simulink model "rx2"  (R2022b)
settings: Solver=FixedStepDiscrete  StartTime=0.0  StopTime=3.3E6  FixedStep=1  RelTol=1e-3  EnableMultiTasking=on
model workspace (MAT data in the model file):
  mwTaskManagerKernelLatency = 0
undefined symbols (not defined in the file or in its folder): Add, jsin, magnitude, rom_pilot_conj_tt, Shift
libraries: hdlsllib x3231, whdlutilities x525, simulink x260, whdlmod x112, whdledac x26, dsphdlmathfun2 x24, commchan3 x1
(part 4 of 59)

== system rx2/process7/OFDM_DEMOD1 ==
  process : Inport
  process_ctrl : Inport  Port=2  OutDataTypeStr=Bus: BUSOFDM1
  Bus Creator : BusCreator  Inputs=8
  Bus Selector : BusSelector  OutputSignals=signal8 (signal 1).valid,signal8 (signal 2).valid,signal8 (signal 3).valid,signal8 (signal 4).valid,signal8 (signal 5).valid,signal8 (signal 6).valid,signal8 (signal 7).valid,signal8 (signal 8).valid
  Demux : Demux  Outputs=8
  Mux : Mux  Inputs=8
  OFDM_demod1 : Subsystem
  OFDM_demod2 : Subsystem
  OFDM_demod3 : Subsystem
  OFDM_demod4 : Subsystem
  OFDM_demod5 : Subsystem
  OFDM_demod6 : Subsystem
  OFDM_demod7 : Subsystem
  OFDM_demod8 : Subsystem
  rxsig : Outport
  Rcrtl_out : Outport  Port=2  OutDataTypeStr=Bus: BUSOFDM1
  wires:
  process_ctrl/1 -> Bus Selector/1
  process/1 -> Demux/1
  Demux/1 -> OFDM_demod1/1(ofdm_sym)
  Demux/2 -> OFDM_demod2/1(ofdm_sym)
  Bus Selector/2 -> OFDM_demod2/2(valid_in)  "<valid>"
  Demux/3 -> OFDM_demod3/1(ofdm_sym)
  Bus Selector/3 -> OFDM_demod3/2(valid_in)  "<valid>"
  Demux/4 -> OFDM_demod4/1(ofdm_sym)
  Bus Selector/4 -> OFDM_demod4/2(valid_in)  "<valid>"
  Bus Selector/5 -> OFDM_demod5/2(valid_in)  "<valid>"
  Bus Selector/6 -> OFDM_demod6/2(valid_in)  "<valid>"
  Bus Selector/7 -> OFDM_demod8/2(valid_in)  "<valid>"
  Bus Selector/8 -> OFDM_demod7/2(valid_in)  "<valid>"
  Demux/5 -> OFDM_demod5/1(ofdm_sym)
  Demux/6 -> OFDM_demod6/1(ofdm_sym)
  Demux/7 -> OFDM_demod8/1(ofdm_sym)
  Demux/8 -> OFDM_demod7/1(ofdm_sym)
  Bus Selector/1 -> OFDM_demod1/2(valid_in)  "<valid>"
  OFDM_demod5/2(ctrl_out) -> Bus Creator/5  "OFDM_ctrl_bf1_process5"
  OFDM_demod2/1(data_out) -> Mux/2
  OFDM_demod7/2(ctrl_out) -> Bus Creator/8  "OFDM_ctrl_bf1_process8"
  OFDM_demod3/1(data_out) -> Mux/3
  OFDM_demod3/2(ctrl_out) -> Bus Creator/3  "OFDM_ctrl_bf1_process3"
  OFDM_demod8/2(ctrl_out) -> Bus Creator/7  "OFDM_ctrl_bf1_process7"
  OFDM_demod5/1(data_out) -> Mux/5
  OFDM_demod1/1(data_out) -> Mux/1
  OFDM_demod2/2(ctrl_out) -> Bus Creator/2  "OFDM_ctrl_bf1_process2"
  OFDM_demod6/2(ctrl_out) -> Bus Creator/6  "OFDM_ctrl_bf1_process6"
  OFDM_demod8/1(data_out) -> Mux/7
  OFDM_demod6/1(data_out) -> Mux/6
  OFDM_demod4/2(ctrl_out) -> Bus Creator/4  "OFDM_ctrl_bf1_process4"
  OFDM_demod1/2(ctrl_out) -> Bus Creator/1  "OFDM_ctrl_bf1_process1"
  OFDM_demod4/1(data_out) -> Mux/4
  OFDM_demod7/1(data_out) -> Mux/8
  Mux/1 -> rxsig/1
  Bus Creator/1 -> Rcrtl_out/1

== system rx2/process7/decoder ==
  chan_est_tt1 : Inport
  port1_ctrl : Inport  Port=2  OutDataTypeStr=Bus: BUSOFDM1
  rxSig_tt1 : Inport  Port=3
  port2_ctrl : Inport  Port=4  OutDataTypeStr=Bus: BUSOFDM1
  nVar_tt : Inport  Port=5  OutDataTypeStr=fixdt(0,16,12)
  Constant2 : Constant  OutDataTypeStr=boolean
  Constant3 : Constant  Value=72  OutDataTypeStr=uint16
  Delay1 : Delay  InitialCondition=0
  Delay2 : Delay  InitialCondition=0
  Detect Rise Positive : hdlsllib/Logic and Bit Operations/Detect Rise Positive  vinit=0  OutDataTypeStr=boolean
  Detect Rise Positive1 : hdlsllib/Logic and Bit Operations/Detect Rise Positive  vinit=0  OutDataTypeStr=boolean
  MRC : Subsystem
  NR CRC Decoder : whdledac/NR CRC Decoder  CRCType=CRC16  FullCheckSum=on  EnableCRCMaskPort=off  SimulateUsing=Code generation
  NR LDPC Decoder : whdledac/NR LDPC Decoder  Algorithm=Min-sum  ScalingFactor=0.75  Termination=Max  SpecifyInputs=Property  NumIterations=15  MaxNumIterations=30  RateCompatible=off  ParityCheckStatus=off  SimulateUsing=Code generation
  Sample Control Bus Selector1 : whdlutilities/Sample Control Bus Selector  OutputSignals=start,end,valid
  deinterleave : Subsystem  mask{length=1584}
      mask prompts: length "the length of data_in"
      mask DialogControl ParameterGroupVar Prompt: 参数
      mask DialogControl Control2 Prompt: the lantency is (length/2+3)
  p-p : Subsystem
  rate recover : Subsystem
  s-p : Subsystem
  soft demodule : Subsystem  mask{demod_length=1584}
      mask prompts: demod_length "The length of demod"
      mask DialogControl ParameterGroupVar Prompt: 参数
      mask DialogControl Control2 Prompt: Latency=4
  synchronization : Subsystem
  synchronize_valid : Subsystem  mask{valid_length=792}
      mask prompts: valid_length "The length of valid"
      mask DialogControl Control2 Prompt: Latency=2
  data_out : Outport
  valid_out : Outport  Port=2
  wires:
  s-p/2(ctrl_out) -> NR LDPC Decoder/2  "ldpc_in_ctrl"
  p-p/1(data) -> NR CRC Decoder/1  "crc_in"
  p-p/2(ctrl) -> NR CRC Decoder/2  "crc_in_ctrl"
  deinterleave/1(data_out) -> rate recover/1(demod)  "deinterleave_data"
  NR LDPC Decoder/2 -> Sample Control Bus Selector1/1  "ldpc_out_ctrl"
  NR LDPC Decoder/1 -> p-p/1(data_in)  "ldpc_out"
  rate recover/1(rate_recover) -> s-p/1(data_in)  "rm_out"
  Detect Rise Positive/1 -> rate recover/3(start_in)
  s-p/1(data_out) -> NR LDPC Decoder/1  "ldpc_in"
  Sample Control Bus Selector1/1 -> p-p/2(start_in)
  Sample Control Bus Selector1/3 -> p-p/3(valid)
  rate recover/4(valid_out) -> s-p/2(valid_in)  "rm_out_valid"
  Constant3/1 -> NR LDPC Decoder/4
  Constant2/1 -> NR LDPC Decoder/3
  deinterleave/2(valid_out) -> rate recover/2(valid_in), Detect Rise Positive/1  "deinterleave_valid"
  synchronization/1(port1_syn) -> Delay2/1
  synchronization/2(port2_syn) -> Delay1/1
  port2_ctrl/1 -> synchronization/4(port2_ctrl)
  rxSig_tt1/1 -> synchronization/2(rxSig_tt)
  port1_ctrl/1 -> synchronization/3(port1_ctrl)
  chan_est_tt1/1 -> synchronization/1(chan_est_tt)
  synchronization/3(valid_syn) -> Detect Rise Positive1/1
  Detect Rise Positive1/1 -> synchronize_valid/1(start)
  Delay2/1 -> MRC/1(chan_est_tt)  "port1"
  Delay1/1 -> MRC/2(rxSig_tt)  "port2"
  synchronize_valid/1(valid_out) -> MRC/3(valid_tt)  "synchronize_valid"
  nVar_tt/1 -> soft demodule/1(nVar_tt)
  MRC/1(G_k_1) -> soft demodule/2(G_k_1)  "G_k_1"
  MRC/2(r_k) -> soft demodule/3(r_k)  "r_k"
  MRC/4(valid) -> soft demodule/5(valid)
  soft demodule/1(demod) -> deinterleave/1(data_tt)  "demod"
  soft demodule/2(valid_out) -> deinterleave/2(valid_tt)  "valid_in"
  MRC/3(start) -> soft demodule/4(start)
  NR CRC Decoder/1 -> data_out/1  "final_data"
  NR CRC Decoder/2 -> valid_out/1  "final_ctrl"

== system rx2/process8/OFDM_DEMOD1 ==
  process : Inport
  process_ctrl : Inport  Port=2  OutDataTypeStr=Bus: BUSOFDM1
  Bus Creator : BusCreator  Inputs=8
  Bus Selector : BusSelector  OutputSignals=signal9 (signal 1).valid,signal9 (signal 2).valid,signal9 (signal 3).valid,signal9 (signal 4).valid,signal9 (signal 5).valid,signal9 (signal 6).valid,signal9 (signal 7).valid,signal9 (signal 8).valid
  Demux : Demux  Outputs=8
  Mux : Mux  Inputs=8
  OFDM_demod1 : Subsystem
  OFDM_demod2 : Subsystem
  OFDM_demod3 : Subsystem
  OFDM_demod4 : Subsystem
  OFDM_demod5 : Subsystem
  OFDM_demod6 : Subsystem
  OFDM_demod7 : Subsystem
  OFDM_demod8 : Subsystem
  rxsig : Outport
  Rcrtl_out : Outport  Port=2  OutDataTypeStr=Bus: BUSOFDM1
  wires:
  Bus Creator/1 -> Rcrtl_out/1
  Mux/1 -> rxsig/1
  OFDM_demod7/1(data_out) -> Mux/8
  OFDM_demod4/1(data_out) -> Mux/4
  OFDM_demod1/2(ctrl_out) -> Bus Creator/1  "OFDM_ctrl_bf1_process1"
  OFDM_demod4/2(ctrl_out) -> Bus Creator/4  "OFDM_ctrl_bf1_process4"
  OFDM_demod6/1(data_out) -> Mux/6
  OFDM_demod8/1(data_out) -> Mux/7
  OFDM_demod6/2(ctrl_out) -> Bus Creator/6  "OFDM_ctrl_bf1_process6"
  OFDM_demod2/2(ctrl_out) -> Bus Creator/2  "OFDM_ctrl_bf1_process2"
  OFDM_demod1/1(data_out) -> Mux/1
  OFDM_demod5/1(data_out) -> Mux/5
  OFDM_demod8/2(ctrl_out) -> Bus Creator/7  "OFDM_ctrl_bf1_process7"
  OFDM_demod3/2(ctrl_out) -> Bus Creator/3  "OFDM_ctrl_bf1_process3"
  OFDM_demod3/1(data_out) -> Mux/3
  OFDM_demod7/2(ctrl_out) -> Bus Creator/8  "OFDM_ctrl_bf1_process8"
  OFDM_demod2/1(data_out) -> Mux/2
  OFDM_demod5/2(ctrl_out) -> Bus Creator/5  "OFDM_ctrl_bf1_process5"
  Bus Selector/1 -> OFDM_demod1/2(valid_in)  "<valid>"
  Demux/8 -> OFDM_demod7/1(ofdm_sym)
  Demux/7 -> OFDM_demod8/1(ofdm_sym)
  Demux/6 -> OFDM_demod6/1(ofdm_sym)
  Demux/5 -> OFDM_demod5/1(ofdm_sym)
  Bus Selector/8 -> OFDM_demod7/2(valid_in)  "<valid>"
  Bus Selector/7 -> OFDM_demod8/2(valid_in)  "<valid>"
  Bus Selector/6 -> OFDM_demod6/2(valid_in)  "<valid>"
  Bus Selector/5 -> OFDM_demod5/2(valid_in)  "<valid>"
  Bus Selector/4 -> OFDM_demod4/2(valid_in)  "<valid>"
  Demux/4 -> OFDM_demod4/1(ofdm_sym)
  Bus Selector/3 -> OFDM_demod3/2(valid_in)  "<valid>"
  Demux/3 -> OFDM_demod3/1(ofdm_sym)
  Bus Selector/2 -> OFDM_demod2/2(valid_in)  "<valid>"
  Demux/2 -> OFDM_demod2/1(ofdm_sym)
  Demux/1 -> OFDM_demod1/1(ofdm_sym)
  process/1 -> Demux/1
  process_ctrl/1 -> Bus Selector/1

== system rx2/process8/decoder ==
  chan_est_tt1 : Inport
  port1_ctrl : Inport  Port=2  OutDataTypeStr=Bus: BUSOFDM1
  rxSig_tt1 : Inport  Port=3
  port2_ctrl : Inport  Port=4  OutDataTypeStr=Bus: BUSOFDM1
  nVar_tt : Inport  Port=5  OutDataTypeStr=fixdt(0,16,12)
  Constant2 : Constant  OutDataTypeStr=boolean
  Constant3 : Constant  Value=72  OutDataTypeStr=uint16
  Delay1 : Delay  InitialCondition=0
  Delay2 : Delay  InitialCondition=0
  Detect Rise Positive : hdlsllib/Logic and Bit Operations/Detect Rise Positive  vinit=0  OutDataTypeStr=boolean
  Detect Rise Positive1 : hdlsllib/Logic and Bit Operations/Detect Rise Positive  vinit=0  OutDataTypeStr=boolean
  MRC : Subsystem
  NR CRC Decoder : whdledac/NR CRC Decoder  CRCType=CRC16  FullCheckSum=on  EnableCRCMaskPort=off  SimulateUsing=Code generation
  NR LDPC Decoder : whdledac/NR LDPC Decoder  Algorithm=Min-sum  ScalingFactor=0.75  Termination=Max  SpecifyInputs=Property  NumIterations=15  MaxNumIterations=30  RateCompatible=off  ParityCheckStatus=off  SimulateUsing=Code generation
  Sample Control Bus Selector1 : whdlutilities/Sample Control Bus Selector  OutputSignals=start,end,valid
  deinterleave : Subsystem  mask{length=1584}
      mask prompts: length "the length of data_in"
      mask DialogControl ParameterGroupVar Prompt: 参数
      mask DialogControl Control2 Prompt: the lantency is (length/2+3)
  p-p : Subsystem
  rate recover : Subsystem
  s-p : Subsystem
  soft demodule : Subsystem  mask{demod_length=1584}
      mask prompts: demod_length "The length of demod"
      mask DialogControl ParameterGroupVar Prompt: 参数
      mask DialogControl Control2 Prompt: Latency=4
  synchronization : Subsystem
  synchronize_valid : Subsystem  mask{valid_length=792}
      mask prompts: valid_length "The length of valid"
      mask DialogControl Control2 Prompt: Latency=2
  data_out : Outport
  valid_out : Outport  Port=2
  wires:
  NR CRC Decoder/2 -> valid_out/1  "final_ctrl"
  NR CRC Decoder/1 -> data_out/1  "final_data"
  MRC/3(start) -> soft demodule/4(start)
  soft demodule/2(valid_out) -> deinterleave/2(valid_tt)  "valid_in"
  soft demodule/1(demod) -> deinterleave/1(data_tt)  "demod"
  MRC/4(valid) -> soft demodule/5(valid)
  MRC/2(r_k) -> soft demodule/3(r_k)  "r_k"
  MRC/1(G_k_1) -> soft demodule/2(G_k_1)  "G_k_1"
  nVar_tt/1 -> soft demodule/1(nVar_tt)
  synchronize_valid/1(valid_out) -> MRC/3(valid_tt)  "synchronize_valid"
  Delay1/1 -> MRC/2(rxSig_tt)  "port2"
  Delay2/1 -> MRC/1(chan_est_tt)  "port1"
  Detect Rise Positive1/1 -> synchronize_valid/1(start)
  synchronization/3(valid_syn) -> Detect Rise Positive1/1
  chan_est_tt1/1 -> synchronization/1(chan_est_tt)
  port1_ctrl/1 -> synchronization/3(port1_ctrl)
  rxSig_tt1/1 -> synchronization/2(rxSig_tt)
  port2_ctrl/1 -> synchronization/4(port2_ctrl)
  synchronization/2(port2_syn) -> Delay1/1
  synchronization/1(port1_syn) -> Delay2/1
  deinterleave/2(valid_out) -> Detect Rise Positive/1, rate recover/2(valid_in)  "deinterleave_valid"
  Constant2/1 -> NR LDPC Decoder/3
  Constant3/1 -> NR LDPC Decoder/4
  rate recover/4(valid_out) -> s-p/2(valid_in)  "rm_out_valid"
  Sample Control Bus Selector1/3 -> p-p/3(valid)
  Sample Control Bus Selector1/1 -> p-p/2(start_in)
  s-p/1(data_out) -> NR LDPC Decoder/1  "ldpc_in"
  Detect Rise Positive/1 -> rate recover/3(start_in)
  rate recover/1(rate_recover) -> s-p/1(data_in)  "rm_out"
  NR LDPC Decoder/1 -> p-p/1(data_in)  "ldpc_out"
  NR LDPC Decoder/2 -> Sample Control Bus Selector1/1  "ldpc_out_ctrl"
  deinterleave/1(data_out) -> rate recover/1(demod)  "deinterleave_data"
  p-p/2(ctrl) -> NR CRC Decoder/2  "crc_in_ctrl"
  p-p/1(data) -> NR CRC Decoder/1  "crc_in"
  s-p/2(ctrl_out) -> NR LDPC Decoder/2  "ldpc_in_ctrl"

== system rx2/process9/OFDM_DEMOD1 ==
  process : Inport
  process_ctrl : Inport  Port=2  OutDataTypeStr=Bus: BUSOFDM1
  Bus Creator : BusCreator  Inputs=8
  Bus Selector : BusSelector  OutputSignals=signal10 (signal 1).valid,signal10 (signal 2).valid,signal10 (signal 3).valid,signal10 (signal 4).valid,signal10 (signal 5).valid,signal10 (signal 6).valid,signal10 (signal 7).valid,signal10 (signal 8).valid
  Demux : Demux  Outputs=8
  Mux : Mux  Inputs=8
  OFDM_demod1 : Subsystem
  OFDM_demod2 : Subsystem
  OFDM_demod3 : Subsystem
  OFDM_demod4 : Subsystem
  OFDM_demod5 : Subsystem
  OFDM_demod6 : Subsystem
  OFDM_demod7 : Subsystem
  OFDM_demod8 : Subsystem
  rxsig : Outport
  Rcrtl_out : Outport  Port=2  OutDataTypeStr=Bus: BUSOFDM1
  wires:
  process_ctrl/1 -> Bus Selector/1
  process/1 -> Demux/1
  Demux/1 -> OFDM_demod1/1(ofdm_sym)
  Demux/2 -> OFDM_demod2/1(ofdm_sym)
  Bus Selector/2 -> OFDM_demod2/2(valid_in)  "<valid>"
  Demux/3 -> OFDM_demod3/1(ofdm_sym)
  Bus Selector/3 -> OFDM_demod3/2(valid_in)  "<valid>"
  Demux/4 -> OFDM_demod4/1(ofdm_sym)
  Bus Selector/4 -> OFDM_demod4/2(valid_in)  "<valid>"
  Bus Selector/5 -> OFDM_demod5/2(valid_in)  "<valid>"
  Bus Selector/6 -> OFDM_demod6/2(valid_in)  "<valid>"
  Bus Selector/7 -> OFDM_demod8/2(valid_in)  "<valid>"
  Bus Selector/8 -> OFDM_demod7/2(valid_in)  "<valid>"
  Demux/5 -> OFDM_demod5/1(ofdm_sym)
  Demux/6 -> OFDM_demod6/1(ofdm_sym)
  Demux/7 -> OFDM_demod8/1(ofdm_sym)
  Demux/8 -> OFDM_demod7/1(ofdm_sym)
  Bus Selector/1 -> OFDM_demod1/2(valid_in)  "<valid>"
  OFDM_demod5/2(ctrl_out) -> Bus Creator/5  "OFDM_ctrl_bf1_process5"
  OFDM_demod2/1(data_out) -> Mux/2
  OFDM_demod7/2(ctrl_out) -> Bus Creator/8  "OFDM_ctrl_bf1_process8"
  OFDM_demod3/1(data_out) -> Mux/3
  OFDM_demod3/2(ctrl_out) -> Bus Creator/3  "OFDM_ctrl_bf1_process3"
  OFDM_demod8/2(ctrl_out) -> Bus Creator/7  "OFDM_ctrl_bf1_process7"
  OFDM_demod5/1(data_out) -> Mux/5
  OFDM_demod1/1(data_out) -> Mux/1
  OFDM_demod2/2(ctrl_out) -> Bus Creator/2  "OFDM_ctrl_bf1_process2"
  OFDM_demod6/2(ctrl_out) -> Bus Creator/6  "OFDM_ctrl_bf1_process6"
  OFDM_demod8/1(data_out) -> Mux/7
  OFDM_demod6/1(data_out) -> Mux/6
  OFDM_demod4/2(ctrl_out) -> Bus Creator/4  "OFDM_ctrl_bf1_process4"
  OFDM_demod1/2(ctrl_out) -> Bus Creator/1  "OFDM_ctrl_bf1_process1"
  OFDM_demod4/1(data_out) -> Mux/4
  OFDM_demod7/1(data_out) -> Mux/8
  Mux/1 -> rxsig/1
  Bus Creator/1 -> Rcrtl_out/1

== system rx2/process9/decoder ==
  chan_est_tt1 : Inport
  port1_ctrl : Inport  Port=2  OutDataTypeStr=Bus: BUSOFDM1
  rxSig_tt1 : Inport  Port=3
  port2_ctrl : Inport  Port=4  OutDataTypeStr=Bus: BUSOFDM1
  nVar_tt : Inport  Port=5  OutDataTypeStr=fixdt(0,16,12)
  Constant2 : Constant  OutDataTypeStr=boolean
  Constant3 : Constant  Value=72  OutDataTypeStr=uint16
  Delay1 : Delay  InitialCondition=0
  Delay2 : Delay  InitialCondition=0
  Detect Rise Positive : hdlsllib/Logic and Bit Operations/Detect Rise Positive  vinit=0  OutDataTypeStr=boolean
  Detect Rise Positive1 : hdlsllib/Logic and Bit Operations/Detect Rise Positive  vinit=0  OutDataTypeStr=boolean
  MRC : Subsystem
  NR CRC Decoder : whdledac/NR CRC Decoder  CRCType=CRC16  FullCheckSum=on  EnableCRCMaskPort=off  SimulateUsing=Code generation
  NR LDPC Decoder : whdledac/NR LDPC Decoder  Algorithm=Min-sum  ScalingFactor=0.75  Termination=Max  SpecifyInputs=Property  NumIterations=15  MaxNumIterations=30  RateCompatible=off  ParityCheckStatus=off  SimulateUsing=Code generation
  Sample Control Bus Selector1 : whdlutilities/Sample Control Bus Selector  OutputSignals=start,end,valid
  deinterleave : Subsystem  mask{length=1584}
      mask prompts: length "the length of data_in"
      mask DialogControl ParameterGroupVar Prompt: 参数
      mask DialogControl Control2 Prompt: the lantency is (length/2+3)
  p-p : Subsystem
  rate recover : Subsystem
  s-p : Subsystem
  soft demodule : Subsystem  mask{demod_length=1584}
      mask prompts: demod_length "The length of demod"
      mask DialogControl ParameterGroupVar Prompt: 参数
      mask DialogControl Control2 Prompt: Latency=4
  synchronization : Subsystem
  synchronize_valid : Subsystem  mask{valid_length=792}
      mask prompts: valid_length "The length of valid"
      mask DialogControl Control2 Prompt: Latency=2
  data_out : Outport
  valid_out : Outport  Port=2
  wires:
  s-p/2(ctrl_out) -> NR LDPC Decoder/2  "ldpc_in_ctrl"
  p-p/1(data) -> NR CRC Decoder/1  "crc_in"
  p-p/2(ctrl) -> NR CRC Decoder/2  "crc_in_ctrl"
  deinterleave/1(data_out) -> rate recover/1(demod)  "deinterleave_data"
  NR LDPC Decoder/2 -> Sample Control Bus Selector1/1  "ldpc_out_ctrl"
  NR LDPC Decoder/1 -> p-p/1(data_in)  "ldpc_out"
  rate recover/1(rate_recover) -> s-p/1(data_in)  "rm_out"
  Detect Rise Positive/1 -> rate recover/3(start_in)
  s-p/1(data_out) -> NR LDPC Decoder/1  "ldpc_in"
  Sample Control Bus Selector1/1 -> p-p/2(start_in)
  Sample Control Bus Selector1/3 -> p-p/3(valid)
  rate recover/4(valid_out) -> s-p/2(valid_in)  "rm_out_valid"
  Constant3/1 -> NR LDPC Decoder/4
  Constant2/1 -> NR LDPC Decoder/3
  deinterleave/2(valid_out) -> rate recover/2(valid_in), Detect Rise Positive/1  "deinterleave_valid"
  synchronization/1(port1_syn) -> Delay2/1
  synchronization/2(port2_syn) -> Delay1/1
  port2_ctrl/1 -> synchronization/4(port2_ctrl)
  rxSig_tt1/1 -> synchronization/2(rxSig_tt)
  port1_ctrl/1 -> synchronization/3(port1_ctrl)
  chan_est_tt1/1 -> synchronization/1(chan_est_tt)
  synchronization/3(valid_syn) -> Detect Rise Positive1/1
  Detect Rise Positive1/1 -> synchronize_valid/1(start)
  Delay2/1 -> MRC/1(chan_est_tt)  "port1"
  Delay1/1 -> MRC/2(rxSig_tt)  "port2"
  synchronize_valid/1(valid_out) -> MRC/3(valid_tt)  "synchronize_valid"
  nVar_tt/1 -> soft demodule/1(nVar_tt)
  MRC/1(G_k_1) -> soft demodule/2(G_k_1)  "G_k_1"
  MRC/2(r_k) -> soft demodule/3(r_k)  "r_k"
  MRC/4(valid) -> soft demodule/5(valid)
  soft demodule/1(demod) -> deinterleave/1(data_tt)  "demod"
  soft demodule/2(valid_out) -> deinterleave/2(valid_tt)  "valid_in"
  MRC/3(start) -> soft demodule/4(start)
  NR CRC Decoder/1 -> data_out/1  "final_data"
  NR CRC Decoder/2 -> valid_out/1  "final_ctrl"

== system rx2/demode1/chan_est1/Subsystem ==
  data_in : Inport
  ctrl_in : Inport  Port=2  OutDataTypeStr=Bus: BUSOFDM1
  HDL_DUT : Subsystem
  HDL_DUT1 : Subsystem
  HDL_DUT2 : Subsystem
  HDL_DUT3 : Subsystem
  HDL_DUT4 : Subsystem
  HDL_DUT5 : Subsystem
  HDL_DUT6 : Subsystem
  HDL_DUT7 : Subsystem
  OFDM_DEMOD1 : Subsystem
  Subsystem1 : Subsystem
  H_out : Outport
  crtl_out : Outport  Port=2  OutDataTypeStr=Bus: BUSOFDM1
  σ²_out : Outport  Port=3
  wires:
  Subsystem1/1(Out1) -> H_out/1
  Subsystem1/3(σ²) -> σ²_out/1
  Subsystem1/2(Out3) -> crtl_out/1
  HDL_DUT/2(w_out) -> Subsystem1/2(w_out)  "w_out"
  HDL_DUT/3(ctrl_out) -> Subsystem1/3(In3)
  HDL_DUT/1(H_out) -> Subsystem1/1(H_out)  "H_out"
  data_in/1 -> OFDM_DEMOD1/1(process)
  OFDM_DEMOD1/1(data_in) -> HDL_DUT/1(data_in)
  ctrl_in/1 -> OFDM_DEMOD1/2(process_ctrl)
  OFDM_DEMOD1/2(OFDM_ctrl_bf1_process1) -> HDL_DUT/2(ctrl_in)
  OFDM_DEMOD1/3(Out3) -> HDL_DUT1/1(data_in)
  OFDM_DEMOD1/4(OFDM_ctrl_bf1_process2) -> HDL_DUT1/2(ctrl_in)
  OFDM_DEMOD1/5(Out5) -> HDL_DUT2/1(data_in)
  OFDM_DEMOD1/6(OFDM_ctrl_bf1_process3) -> HDL_DUT2/2(ctrl_in)
  OFDM_DEMOD1/7(Out7) -> HDL_DUT3/1(data_in)
  OFDM_DEMOD1/8(OFDM_ctrl_bf1_process4) -> HDL_DUT3/2(ctrl_in)
  OFDM_DEMOD1/9(Out9) -> HDL_DUT4/1(data_in)
  OFDM_DEMOD1/10(OFDM_ctrl_bf1_process5) -> HDL_DUT4/2(ctrl_in)
  OFDM_DEMOD1/11(Out11) -> HDL_DUT5/1(data_in)
  OFDM_DEMOD1/12(OFDM_ctrl_bf1_process6) -> HDL_DUT5/2(ctrl_in)
  OFDM_DEMOD1/13(Out13) -> HDL_DUT6/1(data_in)
  OFDM_DEMOD1/14(OFDM_ctrl_bf1_process7) -> HDL_DUT6/2(ctrl_in)
  OFDM_DEMOD1/15(Out15) -> HDL_DUT7/1(data_in)
  OFDM_DEMOD1/16(OFDM_ctrl_bf1_process8) -> HDL_DUT7/2(ctrl_in)
  HDL_DUT1/1(H_out) -> Subsystem1/4(H_out1)  "H_out"
  HDL_DUT1/2(w_out) -> Subsystem1/5(w_out1)  "w_out"
  HDL_DUT1/3(ctrl_out) -> Subsystem1/6(ctrl_out)
  HDL_DUT2/1(H_out) -> Subsystem1/7(H_out2)  "H_out"
  HDL_DUT2/2(w_out) -> Subsystem1/8(w_out2)  "w_out"
  HDL_DUT2/3(ctrl_out) -> Subsystem1/9(In9)
  HDL_DUT3/1(H_out) -> Subsystem1/10(H_out3)  "H_out"
  HDL_DUT3/2(w_out) -> Subsystem1/11(w_out3)  "w_out"
  HDL_DUT3/3(ctrl_out) -> Subsystem1/12(In12)
  HDL_DUT4/1(H_out) -> Subsystem1/13(H_out4)  "H_out"
  HDL_DUT4/2(w_out) -> Subsystem1/14(w_out4)  "w_out"
  HDL_DUT4/3(ctrl_out) -> Subsystem1/15(In15)
  HDL_DUT5/1(H_out) -> Subsystem1/16(H_out5)  "H_out"
  HDL_DUT5/2(w_out) -> Subsystem1/17(w_out5)  "w_out"
  HDL_DUT5/3(ctrl_out) -> Subsystem1/18(In18)
  HDL_DUT6/1(H_out) -> Subsystem1/19(H_out6)  "H_out"
  HDL_DUT6/2(w_out) -> Subsystem1/20(w_out6)  "w_out"
  HDL_DUT6/3(ctrl_out) -> Subsystem1/21(In21)
  HDL_DUT7/1(H_out) -> Subsystem1/22(H_out7)  "H_out"
  HDL_DUT7/2(w_out) -> Subsystem1/23(w_out7)  "w_out"
  HDL_DUT7/3(ctrl_out) -> Subsystem1/24(In24)

== system rx2/process divide/transport_block1/Subsystem1 ==
  data_in : Inport
  select_valid : Inport  Port=2  OutDataTypeStr=boolean
  Constant : Constant  Value=0  OutDataTypeStr=fixdt(1,16,14)
  Real-Imag to Complex : RealImagToComplex
  Switch : Switch  Criteria=u2 ~= 0  SaturateOnIntegerOverflow=off  InputSameDT=off
  ctrl_gen : Subsystem
  data_out : Outport
  ctrl_out : Outport  Port=2
  wires:
  Switch/1 -> ctrl_gen/1(data_in)
  Constant/1 -> Real-Imag to Complex/2, Real-Imag to Complex/1
  select_valid/1 -> ctrl_gen/2(valid_in), Switch/2
  ctrl_gen/1(data_out) -> data_out/1
  ctrl_gen/2(ctrl_out) -> ctrl_out/1
  data_in/1 -> Switch/1
  Real-Imag to Complex/1 -> Switch/3

== system rx2/process divide/transport_block1/Subsystem10 ==
  data_in : Inport
  select_valid : Inport  Port=2  OutDataTypeStr=boolean
  Constant : Constant  Value=0  OutDataTypeStr=fixdt(1,16,14)
  Real-Imag to Complex : RealImagToComplex
  Switch : Switch  Criteria=u2 ~= 0  SaturateOnIntegerOverflow=off  InputSameDT=off
  ctrl_gen : Subsystem
  data_out : Outport
  ctrl_out : Outport  Port=2
  wires:
  Real-Imag to Complex/1 -> Switch/3
  data_in/1 -> Switch/1
  ctrl_gen/2(ctrl_out) -> ctrl_out/1
  ctrl_gen/1(data_out) -> data_out/1
  select_valid/1 -> Switch/2, ctrl_gen/2(valid_in)
  Constant/1 -> Real-Imag to Complex/1, Real-Imag to Complex/2
  Switch/1 -> ctrl_gen/1(data_in)

== system rx2/process divide/transport_block1/Subsystem11 ==
  data_in : Inport
  select_valid : Inport  Port=2  OutDataTypeStr=boolean
  Constant : Constant  Value=0  OutDataTypeStr=fixdt(1,16,14)
  Real-Imag to Complex : RealImagToComplex
  Switch : Switch  Criteria=u2 ~= 0  SaturateOnIntegerOverflow=off  InputSameDT=off
  ctrl_gen : Subsystem
  data_out : Outport
  ctrl_out : Outport  Port=2
  wires:
  Real-Imag to Complex/1 -> Switch/3
  data_in/1 -> Switch/1
  ctrl_gen/2(ctrl_out) -> ctrl_out/1
  ctrl_gen/1(data_out) -> data_out/1
  select_valid/1 -> Switch/2, ctrl_gen/2(valid_in)
  Constant/1 -> Real-Imag to Complex/1, Real-Imag to Complex/2
  Switch/1 -> ctrl_gen/1(data_in)

== system rx2/process divide/transport_block1/Subsystem12 ==
  data_in : Inport
  select_valid : Inport  Port=2  OutDataTypeStr=boolean
  Constant : Constant  Value=0  OutDataTypeStr=fixdt(1,16,14)
  Real-Imag to Complex : RealImagToComplex
  Switch : Switch  Criteria=u2 ~= 0  SaturateOnIntegerOverflow=off  InputSameDT=off
  ctrl_gen : Subsystem
  data_out : Outport
  ctrl_out : Outport  Port=2
  wires:
  Real-Imag to Complex/1 -> Switch/3
  data_in/1 -> Switch/1
  ctrl_gen/2(ctrl_out) -> ctrl_out/1
  ctrl_gen/1(data_out) -> data_out/1
  select_valid/1 -> Switch/2, ctrl_gen/2(valid_in)
  Constant/1 -> Real-Imag to Complex/1, Real-Imag to Complex/2
  Switch/1 -> ctrl_gen/1(data_in)

== system rx2/process divide/transport_block1/Subsystem13 ==
  data_in : Inport
  select_valid : Inport  Port=2  OutDataTypeStr=boolean
  Constant : Constant  Value=0  OutDataTypeStr=fixdt(1,16,14)
  Real-Imag to Complex : RealImagToComplex
  Switch : Switch  Criteria=u2 ~= 0  SaturateOnIntegerOverflow=off  InputSameDT=off
  ctrl_gen : Subsystem
  data_out : Outport
  ctrl_out : Outport  Port=2
  wires:
  Real-Imag to Complex/1 -> Switch/3
  data_in/1 -> Switch/1
  ctrl_gen/2(ctrl_out) -> ctrl_out/1
  ctrl_gen/1(data_out) -> data_out/1
  select_valid/1 -> Switch/2, ctrl_gen/2(valid_in)
  Constant/1 -> Real-Imag to Complex/1, Real-Imag to Complex/2
  Switch/1 -> ctrl_gen/1(data_in)

== system rx2/process divide/transport_block1/Subsystem14 ==
  data_in : Inport
  select_valid : Inport  Port=2  OutDataTypeStr=boolean
  Constant : Constant  Value=0  OutDataTypeStr=fixdt(1,16,14)
  Real-Imag to Complex : RealImagToComplex
  Switch : Switch  Criteria=u2 ~= 0  SaturateOnIntegerOverflow=off  InputSameDT=off
  ctrl_gen : Subsystem
  data_out : Outport
  ctrl_out : Outport  Port=2
  wires:
  Real-Imag to Complex/1 -> Switch/3
  data_in/1 -> Switch/1
  ctrl_gen/2(ctrl_out) -> ctrl_out/1
  ctrl_gen/1(data_out) -> data_out/1
  select_valid/1 -> Switch/2, ctrl_gen/2(valid_in)
  Constant/1 -> Real-Imag to Complex/1, Real-Imag to Complex/2
  Switch/1 -> ctrl_gen/1(data_in)

== system rx2/process divide/transport_block1/Subsystem2 ==
  data_in : Inport
  select_valid : Inport  Port=2  OutDataTypeStr=boolean
  Constant : Constant  Value=0  OutDataTypeStr=fixdt(1,16,14)
  Real-Imag to Complex : RealImagToComplex
  Switch : Switch  Criteria=u2 ~= 0  SaturateOnIntegerOverflow=off  InputSameDT=off
  ctrl_gen : Subsystem
  data_out : Outport
  ctrl_out : Outport  Port=2
  wires:
  Real-Imag to Complex/1 -> Switch/3
  data_in/1 -> Switch/1
  ctrl_gen/2(ctrl_out) -> ctrl_out/1
  ctrl_gen/1(data_out) -> data_out/1
  select_valid/1 -> Switch/2, ctrl_gen/2(valid_in)
  Constant/1 -> Real-Imag to Complex/1, Real-Imag to Complex/2
  Switch/1 -> ctrl_gen/1(data_in)

== system rx2/process divide/transport_block1/Subsystem3 ==
  data_in : Inport
  select_valid : Inport  Port=2  OutDataTypeStr=boolean
  Constant : Constant  Value=0  OutDataTypeStr=fixdt(1,16,14)
  Real-Imag to Complex : RealImagToComplex
  Switch : Switch  Criteria=u2 ~= 0  SaturateOnIntegerOverflow=off  InputSameDT=off
  ctrl_gen : Subsystem
  data_out : Outport
  ctrl_out : Outport  Port=2
  wires:
  Switch/1 -> ctrl_gen/1(data_in)
  Constant/1 -> Real-Imag to Complex/2, Real-Imag to Complex/1
  select_valid/1 -> ctrl_gen/2(valid_in), Switch/2
  ctrl_gen/1(data_out) -> data_out/1
  ctrl_gen/2(ctrl_out) -> ctrl_out/1
  data_in/1 -> Switch/1
  Real-Imag to Complex/1 -> Switch/3

== system rx2/process divide/transport_block1/Subsystem4 ==
  data_in : Inport
  select_valid : Inport  Port=2  OutDataTypeStr=boolean
  Constant : Constant  Value=0  OutDataTypeStr=fixdt(1,16,14)
  Real-Imag to Complex : RealImagToComplex
  Switch : Switch  Criteria=u2 ~= 0  SaturateOnIntegerOverflow=off  InputSameDT=off
  ctrl_gen : Subsystem
  data_out : Outport
  ctrl_out : Outport  Port=2
  wires:
  Real-Imag to Complex/1 -> Switch/3
  data_in/1 -> Switch/1
  ctrl_gen/2(ctrl_out) -> ctrl_out/1
  ctrl_gen/1(data_out) -> data_out/1
  select_valid/1 -> Switch/2, ctrl_gen/2(valid_in)
  Constant/1 -> Real-Imag to Complex/1, Real-Imag to Complex/2
  Switch/1 -> ctrl_gen/1(data_in)

== system rx2/process divide/transport_block1/Subsystem5 ==
  data_in : Inport
  select_valid : Inport  Port=2  OutDataTypeStr=boolean
  Constant : Constant  Value=0  OutDataTypeStr=fixdt(1,16,14)
  Real-Imag to Complex : RealImagToComplex
  Switch : Switch  Criteria=u2 ~= 0  SaturateOnIntegerOverflow=off  InputSameDT=off
  ctrl_gen : Subsystem
  data_out : Outport
  ctrl_out : Outport  Port=2
  wires:
  Real-Imag to Complex/1 -> Switch/3
  data_in/1 -> Switch/1
  ctrl_gen/2(ctrl_out) -> ctrl_out/1
  ctrl_gen/1(data_out) -> data_out/1
  select_valid/1 -> Switch/2, ctrl_gen/2(valid_in)
  Constant/1 -> Real-Imag to Complex/1, Real-Imag to Complex/2
  Switch/1 -> ctrl_gen/1(data_in)

== system rx2/process divide/transport_block1/Subsystem6 ==
  data_in : Inport
  select_valid : Inport  Port=2  OutDataTypeStr=boolean
  Constant : Constant  Value=0  OutDataTypeStr=fixdt(1,16,14)
  Real-Imag to Complex : RealImagToComplex
  Switch : Switch  Criteria=u2 ~= 0  SaturateOnIntegerOverflow=off  InputSameDT=off
  ctrl_gen : Subsystem
  data_out : Outport
  ctrl_out : Outport  Port=2
  wires:
  Real-Imag to Complex/1 -> Switch/3
  data_in/1 -> Switch/1
  ctrl_gen/2(ctrl_out) -> ctrl_out/1
  ctrl_gen/1(data_out) -> data_out/1
  select_valid/1 -> Switch/2, ctrl_gen/2(valid_in)
  Constant/1 -> Real-Imag to Complex/1, Real-Imag to Complex/2
  Switch/1 -> ctrl_gen/1(data_in)

== system rx2/process divide/transport_block1/Subsystem7 ==
  data_in : Inport
  select_valid : Inport  Port=2  OutDataTypeStr=boolean
  Constant : Constant  Value=0  OutDataTypeStr=fixdt(1,16,14)
  Real-Imag to Complex : RealImagToComplex
  Switch : Switch  Criteria=u2 ~= 0  SaturateOnIntegerOverflow=off  InputSameDT=off
  ctrl_gen : Subsystem
  data_out : Outport
  ctrl_out : Outport  Port=2
  wires:
  Real-Imag to Complex/1 -> Switch/3
  data_in/1 -> Switch/1
  ctrl_gen/2(ctrl_out) -> ctrl_out/1
  ctrl_gen/1(data_out) -> data_out/1
  select_valid/1 -> Switch/2, ctrl_gen/2(valid_in)
  Constant/1 -> Real-Imag to Complex/1, Real-Imag to Complex/2
  Switch/1 -> ctrl_gen/1(data_in)

== system rx2/process divide/transport_block1/Subsystem8 ==
  data_in : Inport
  select_valid : Inport  Port=2  OutDataTypeStr=boolean
  Constant : Constant  Value=0  OutDataTypeStr=fixdt(1,16,14)
  Real-Imag to Complex : RealImagToComplex
  Switch : Switch  Criteria=u2 ~= 0  SaturateOnIntegerOverflow=off  InputSameDT=off
  ctrl_gen : Subsystem
  data_out : Outport
  ctrl_out : Outport  Port=2
  wires:
  Real-Imag to Complex/1 -> Switch/3
  data_in/1 -> Switch/1
  ctrl_gen/2(ctrl_out) -> ctrl_out/1
  ctrl_gen/1(data_out) -> data_out/1
  select_valid/1 -> Switch/2, ctrl_gen/2(valid_in)
  Constant/1 -> Real-Imag to Complex/1, Real-Imag to Complex/2
  Switch/1 -> ctrl_gen/1(data_in)

== system rx2/process divide/transport_block1/Subsystem9 ==
  data_in : Inport
  select_valid : Inport  Port=2  OutDataTypeStr=boolean
  Constant : Constant  Value=0  OutDataTypeStr=fixdt(1,16,14)
  Real-Imag to Complex : RealImagToComplex
  Switch : Switch  Criteria=u2 ~= 0  SaturateOnIntegerOverflow=off  InputSameDT=off
  ctrl_gen : Subsystem
  data_out : Outport
  ctrl_out : Outport  Port=2
  wires:
  Real-Imag to Complex/1 -> Switch/3
  data_in/1 -> Switch/1
  ctrl_gen/2(ctrl_out) -> ctrl_out/1
  ctrl_gen/1(data_out) -> data_out/1
  select_valid/1 -> Switch/2, ctrl_gen/2(valid_in)
  Constant/1 -> Real-Imag to Complex/1, Real-Imag to Complex/2
  Switch/1 -> ctrl_gen/1(data_in)

== system rx2/process divide/transport_block2/Subsystem1 ==
  data_in : Inport
  select_valid : Inport  Port=2  OutDataTypeStr=boolean
  Constant : Constant  Value=0  OutDataTypeStr=fixdt(1,16,14)
  Real-Imag to Complex : RealImagToComplex
  Switch : Switch  Criteria=u2 ~= 0  SaturateOnIntegerOverflow=off  InputSameDT=off
  ctrl_gen : Subsystem
  data_out : Outport
  ctrl_out : Outport  Port=2
  wires:
  Real-Imag to Complex/1 -> Switch/3
  data_in/1 -> Switch/1
  ctrl_gen/2(ctrl_out) -> ctrl_out/1
  ctrl_gen/1(data_out) -> data_out/1
  select_valid/1 -> Switch/2, ctrl_gen/2(valid_in)
  Constant/1 -> Real-Imag to Complex/1, Real-Imag to Complex/2
  Switch/1 -> ctrl_gen/1(data_in)

== system rx2/process divide/transport_block2/Subsystem10 ==
  data_in : Inport
  select_valid : Inport  Port=2  OutDataTypeStr=boolean
  Constant : Constant  Value=0  OutDataTypeStr=fixdt(1,16,14)
  Real-Imag to Complex : RealImagToComplex
  Switch : Switch  Criteria=u2 ~= 0  SaturateOnIntegerOverflow=off  InputSameDT=off
  ctrl_gen : Subsystem
  data_out : Outport
  ctrl_out : Outport  Port=2
  wires:
  Switch/1 -> ctrl_gen/1(data_in)
  Constant/1 -> Real-Imag to Complex/2, Real-Imag to Complex/1
  select_valid/1 -> ctrl_gen/2(valid_in), Switch/2
  ctrl_gen/1(data_out) -> data_out/1
  ctrl_gen/2(ctrl_out) -> ctrl_out/1
  data_in/1 -> Switch/1
  Real-Imag to Complex/1 -> Switch/3

== system rx2/process divide/transport_block2/Subsystem11 ==
  data_in : Inport
  select_valid : Inport  Port=2  OutDataTypeStr=boolean
  Constant : Constant  Value=0  OutDataTypeStr=fixdt(1,16,14)
  Real-Imag to Complex : RealImagToComplex
  Switch : Switch  Criteria=u2 ~= 0  SaturateOnIntegerOverflow=off  InputSameDT=off
  ctrl_gen : Subsystem
  data_out : Outport
  ctrl_out : Outport  Port=2
  wires:
  Switch/1 -> ctrl_gen/1(data_in)
  Constant/1 -> Real-Imag to Complex/2, Real-Imag to Complex/1
  select_valid/1 -> ctrl_gen/2(valid_in), Switch/2
  ctrl_gen/1(data_out) -> data_out/1
  ctrl_gen/2(ctrl_out) -> ctrl_out/1
  data_in/1 -> Switch/1
  Real-Imag to Complex/1 -> Switch/3

== system rx2/process divide/transport_block2/Subsystem12 ==
  data_in : Inport
  select_valid : Inport  Port=2  OutDataTypeStr=boolean
  Constant : Constant  Value=0  OutDataTypeStr=fixdt(1,16,14)
  Real-Imag to Complex : RealImagToComplex
  Switch : Switch  Criteria=u2 ~= 0  SaturateOnIntegerOverflow=off  InputSameDT=off
  ctrl_gen : Subsystem
  data_out : Outport
  ctrl_out : Outport  Port=2
  wires:
  Switch/1 -> ctrl_gen/1(data_in)
  Constant/1 -> Real-Imag to Complex/2, Real-Imag to Complex/1
  select_valid/1 -> ctrl_gen/2(valid_in), Switch/2
  ctrl_gen/1(data_out) -> data_out/1
  ctrl_gen/2(ctrl_out) -> ctrl_out/1
  data_in/1 -> Switch/1
  Real-Imag to Complex/1 -> Switch/3

== system rx2/process divide/transport_block2/Subsystem13 ==
  data_in : Inport
  select_valid : Inport  Port=2  OutDataTypeStr=boolean
  Constant : Constant  Value=0  OutDataTypeStr=fixdt(1,16,14)
  Real-Imag to Complex : RealImagToComplex
  Switch : Switch  Criteria=u2 ~= 0  SaturateOnIntegerOverflow=off  InputSameDT=off
  ctrl_gen : Subsystem
  data_out : Outport
  ctrl_out : Outport  Port=2
  wires:
  Switch/1 -> ctrl_gen/1(data_in)
  Constant/1 -> Real-Imag to Complex/2, Real-Imag to Complex/1
  select_valid/1 -> ctrl_gen/2(valid_in), Switch/2
  ctrl_gen/1(data_out) -> data_out/1
  ctrl_gen/2(ctrl_out) -> ctrl_out/1
  data_in/1 -> Switch/1
  Real-Imag to Complex/1 -> Switch/3

== system rx2/process divide/transport_block2/Subsystem14 ==
  data_in : Inport
  select_valid : Inport  Port=2  OutDataTypeStr=boolean
  Constant : Constant  Value=0  OutDataTypeStr=fixdt(1,16,14)
  Real-Imag to Complex : RealImagToComplex
  Switch : Switch  Criteria=u2 ~= 0  SaturateOnIntegerOverflow=off  InputSameDT=off
  ctrl_gen : Subsystem
  data_out : Outport
  ctrl_out : Outport  Port=2
  wires:
  Switch/1 -> ctrl_gen/1(data_in)
  Constant/1 -> Real-Imag to Complex/2, Real-Imag to Complex/1
  select_valid/1 -> ctrl_gen/2(valid_in), Switch/2
  ctrl_gen/1(data_out) -> data_out/1
  ctrl_gen/2(ctrl_out) -> ctrl_out/1
  data_in/1 -> Switch/1
  Real-Imag to Complex/1 -> Switch/3

== system rx2/process divide/transport_block2/Subsystem2 ==
  data_in : Inport
  select_valid : Inport  Port=2  OutDataTypeStr=boolean
  Constant : Constant  Value=0  OutDataTypeStr=fixdt(1,16,14)
  Real-Imag to Complex : RealImagToComplex
  Switch : Switch  Criteria=u2 ~= 0  SaturateOnIntegerOverflow=off  InputSameDT=off
  ctrl_gen : Subsystem
  data_out : Outport
  ctrl_out : Outport  Port=2
  wires:
  Switch/1 -> ctrl_gen/1(data_in)
  Constant/1 -> Real-Imag to Complex/2, Real-Imag to Complex/1
  select_valid/1 -> ctrl_gen/2(valid_in), Switch/2
  ctrl_gen/1(data_out) -> data_out/1
  ctrl_gen/2(ctrl_out) -> ctrl_out/1
  data_in/1 -> Switch/1
  Real-Imag to Complex/1 -> Switch/3

== system rx2/process divide/transport_block2/Subsystem3 ==
  data_in : Inport
  select_valid : Inport  Port=2  OutDataTypeStr=boolean
  Constant : Constant  Value=0  OutDataTypeStr=fixdt(1,16,14)
  Real-Imag to Complex : RealImagToComplex
  Switch : Switch  Criteria=u2 ~= 0  SaturateOnIntegerOverflow=off  InputSameDT=off
  ctrl_gen : Subsystem
  data_out : Outport
  ctrl_out : Outport  Port=2
  wires:
  Real-Imag to Complex/1 -> Switch/3
  data_in/1 -> Switch/1
  ctrl_gen/2(ctrl_out) -> ctrl_out/1
  ctrl_gen/1(data_out) -> data_out/1
  select_valid/1 -> Switch/2, ctrl_gen/2(valid_in)
  Constant/1 -> Real-Imag to Complex/1, Real-Imag to Complex/2
  Switch/1 -> ctrl_gen/1(data_in)

== system rx2/process divide/transport_block2/Subsystem4 ==
  data_in : Inport
  select_valid : Inport  Port=2  OutDataTypeStr=boolean
  Constant : Constant  Value=0  OutDataTypeStr=fixdt(1,16,14)
  Real-Imag to Complex : RealImagToComplex
  Switch : Switch  Criteria=u2 ~= 0  SaturateOnIntegerOverflow=off  InputSameDT=off
  ctrl_gen : Subsystem
  data_out : Outport
  ctrl_out : Outport  Port=2
  wires:
  Switch/1 -> ctrl_gen/1(data_in)
  Constant/1 -> Real-Imag to Complex/2, Real-Imag to Complex/1
  select_valid/1 -> ctrl_gen/2(valid_in), Switch/2
  ctrl_gen/1(data_out) -> data_out/1
  ctrl_gen/2(ctrl_out) -> ctrl_out/1
  data_in/1 -> Switch/1
  Real-Imag to Complex/1 -> Switch/3

== system rx2/process divide/transport_block2/Subsystem5 ==
  data_in : Inport
  select_valid : Inport  Port=2  OutDataTypeStr=boolean
  Constant : Constant  Value=0  OutDataTypeStr=fixdt(1,16,14)
  Real-Imag to Complex : RealImagToComplex
  Switch : Switch  Criteria=u2 ~= 0  SaturateOnIntegerOverflow=off  InputSameDT=off
  ctrl_gen : Subsystem
  data_out : Outport
  ctrl_out : Outport  Port=2
  wires:
  Switch/1 -> ctrl_gen/1(data_in)
  Constant/1 -> Real-Imag to Complex/2, Real-Imag to Complex/1
  select_valid/1 -> ctrl_gen/2(valid_in), Switch/2
  ctrl_gen/1(data_out) -> data_out/1
  ctrl_gen/2(ctrl_out) -> ctrl_out/1
  data_in/1 -> Switch/1
  Real-Imag to Complex/1 -> Switch/3

== system rx2/process divide/transport_block2/Subsystem6 ==
  data_in : Inport
  select_valid : Inport  Port=2  OutDataTypeStr=boolean
  Constant : Constant  Value=0  OutDataTypeStr=fixdt(1,16,14)
  Real-Imag to Complex : RealImagToComplex
  Switch : Switch  Criteria=u2 ~= 0  SaturateOnIntegerOverflow=off  InputSameDT=off
  ctrl_gen : Subsystem
  data_out : Outport
  ctrl_out : Outport  Port=2
  wires:
  Switch/1 -> ctrl_gen/1(data_in)
  Constant/1 -> Real-Imag to Complex/2, Real-Imag to Complex/1
  select_valid/1 -> ctrl_gen/2(valid_in), Switch/2
  ctrl_gen/1(data_out) -> data_out/1
  ctrl_gen/2(ctrl_out) -> ctrl_out/1
  data_in/1 -> Switch/1
  Real-Imag to Complex/1 -> Switch/3

== system rx2/process divide/transport_block2/Subsystem7 ==
  data_in : Inport
  select_valid : Inport  Port=2  OutDataTypeStr=boolean
  Constant : Constant  Value=0  OutDataTypeStr=fixdt(1,16,14)
  Real-Imag to Complex : RealImagToComplex
  Switch : Switch  Criteria=u2 ~= 0  SaturateOnIntegerOverflow=off  InputSameDT=off
  ctrl_gen : Subsystem
  data_out : Outport
  ctrl_out : Outport  Port=2
  wires:
  Switch/1 -> ctrl_gen/1(data_in)
  Constant/1 -> Real-Imag to Complex/2, Real-Imag to Complex/1
  select_valid/1 -> ctrl_gen/2(valid_in), Switch/2
  ctrl_gen/1(data_out) -> data_out/1
  ctrl_gen/2(ctrl_out) -> ctrl_out/1
  data_in/1 -> Switch/1
  Real-Imag to Complex/1 -> Switch/3

== system rx2/process divide/transport_block2/Subsystem8 ==
  data_in : Inport
  select_valid : Inport  Port=2  OutDataTypeStr=boolean
  Constant : Constant  Value=0  OutDataTypeStr=fixdt(1,16,14)
  Real-Imag to Complex : RealImagToComplex
  Switch : Switch  Criteria=u2 ~= 0  SaturateOnIntegerOverflow=off  InputSameDT=off
  ctrl_gen : Subsystem
  data_out : Outport
  ctrl_out : Outport  Port=2
  wires:
  Switch/1 -> ctrl_gen/1(data_in)
  Constant/1 -> Real-Imag to Complex/2, Real-Imag to Complex/1
  select_valid/1 -> ctrl_gen/2(valid_in), Switch/2
  ctrl_gen/1(data_out) -> data_out/1
  ctrl_gen/2(ctrl_out) -> ctrl_out/1
  data_in/1 -> Switch/1
  Real-Imag to Complex/1 -> Switch/3

== system rx2/process divide/transport_block2/Subsystem9 ==
  data_in : Inport
  select_valid : Inport  Port=2  OutDataTypeStr=boolean
  Constant : Constant  Value=0  OutDataTypeStr=fixdt(1,16,14)
  Real-Imag to Complex : RealImagToComplex
  Switch : Switch  Criteria=u2 ~= 0  SaturateOnIntegerOverflow=off  InputSameDT=off
  ctrl_gen : Subsystem
  data_out : Outport
  ctrl_out : Outport  Port=2
  wires:
  Switch/1 -> ctrl_gen/1(data_in)
  Constant/1 -> Real-Imag to Complex/2, Real-Imag to Complex/1
  select_valid/1 -> ctrl_gen/2(valid_in), Switch/2
  ctrl_gen/1(data_out) -> data_out/1
  ctrl_gen/2(ctrl_out) -> ctrl_out/1
  data_in/1 -> Switch/1
  Real-Imag to Complex/1 -> Switch/3

== system rx2/process divide/transport_block3/Subsystem1 ==
  data_in : Inport
  select_valid : Inport  Port=2  OutDataTypeStr=boolean
  Constant : Constant  Value=0  OutDataTypeStr=fixdt(1,16,14)
  Real-Imag to Complex : RealImagToComplex
  Switch : Switch  Criteria=u2 ~= 0  SaturateOnIntegerOverflow=off  InputSameDT=off
  ctrl_gen : Subsystem
  data_out : Outport
  ctrl_out : Outport  Port=2
  wires:
  Switch/1 -> ctrl_gen/1(data_in)
  Constant/1 -> Real-Imag to Complex/2, Real-Imag to Complex/1
  select_valid/1 -> ctrl_gen/2(valid_in), Switch/2
  ctrl_gen/1(data_out) -> data_out/1
  ctrl_gen/2(ctrl_out) -> ctrl_out/1
  data_in/1 -> Switch/1
  Real-Imag to Complex/1 -> Switch/3

== system rx2/process divide/transport_block3/Subsystem10 ==
  data_in : Inport
  select_valid : Inport  Port=2  OutDataTypeStr=boolean
  Constant : Constant  Value=0  OutDataTypeStr=fixdt(1,16,14)
  Real-Imag to Complex : RealImagToComplex
  Switch : Switch  Criteria=u2 ~= 0  SaturateOnIntegerOverflow=off  InputSameDT=off
  ctrl_gen : Subsystem
  data_out : Outport
  ctrl_out : Outport  Port=2
  wires:
  Real-Imag to Complex/1 -> Switch/3
  data_in/1 -> Switch/1
  ctrl_gen/2(ctrl_out) -> ctrl_out/1
  ctrl_gen/1(data_out) -> data_out/1
  select_valid/1 -> Switch/2, ctrl_gen/2(valid_in)
  Constant/1 -> Real-Imag to Complex/1, Real-Imag to Complex/2
  Switch/1 -> ctrl_gen/1(data_in)

== system rx2/process divide/transport_block3/Subsystem11 ==
  data_in : Inport
  select_valid : Inport  Port=2  OutDataTypeStr=boolean
  Constant : Constant  Value=0  OutDataTypeStr=fixdt(1,16,14)
  Real-Imag to Complex : RealImagToComplex
  Switch : Switch  Criteria=u2 ~= 0  SaturateOnIntegerOverflow=off  InputSameDT=off
  ctrl_gen : Subsystem
  data_out : Outport
  ctrl_out : Outport  Port=2
  wires:
  Real-Imag to Complex/1 -> Switch/3
  data_in/1 -> Switch/1
  ctrl_gen/2(ctrl_out) -> ctrl_out/1
  ctrl_gen/1(data_out) -> data_out/1
  select_valid/1 -> Switch/2, ctrl_gen/2(valid_in)
  Constant/1 -> Real-Imag to Complex/1, Real-Imag to Complex/2
  Switch/1 -> ctrl_gen/1(data_in)

== system rx2/process divide/transport_block3/Subsystem12 ==
  data_in : Inport
  select_valid : Inport  Port=2  OutDataTypeStr=boolean
  Constant : Constant  Value=0  OutDataTypeStr=fixdt(1,16,14)
  Real-Imag to Complex : RealImagToComplex
  Switch : Switch  Criteria=u2 ~= 0  SaturateOnIntegerOverflow=off  InputSameDT=off
  ctrl_gen : Subsystem
  data_out : Outport
  ctrl_out : Outport  Port=2
  wires:
  Real-Imag to Complex/1 -> Switch/3
  data_in/1 -> Switch/1
  ctrl_gen/2(ctrl_out) -> ctrl_out/1
  ctrl_gen/1(data_out) -> data_out/1
  select_valid/1 -> Switch/2, ctrl_gen/2(valid_in)
  Constant/1 -> Real-Imag to Complex/1, Real-Imag to Complex/2
  Switch/1 -> ctrl_gen/1(data_in)

== system rx2/process divide/transport_block3/Subsystem13 ==
  data_in : Inport
  select_valid : Inport  Port=2  OutDataTypeStr=boolean
  Constant : Constant  Value=0  OutDataTypeStr=fixdt(1,16,14)
  Real-Imag to Complex : RealImagToComplex
  Switch : Switch  Criteria=u2 ~= 0  SaturateOnIntegerOverflow=off  InputSameDT=off
  ctrl_gen : Subsystem
  data_out : Outport
  ctrl_out : Outport  Port=2
  wires:
  Real-Imag to Complex/1 -> Switch/3
  data_in/1 -> Switch/1
  ctrl_gen/2(ctrl_out) -> ctrl_out/1
  ctrl_gen/1(data_out) -> data_out/1
  select_valid/1 -> Switch/2, ctrl_gen/2(valid_in)
  Constant/1 -> Real-Imag to Complex/1, Real-Imag to Complex/2
  Switch/1 -> ctrl_gen/1(data_in)

== system rx2/process divide/transport_block3/Subsystem14 ==
  data_in : Inport
  select_valid : Inport  Port=2  OutDataTypeStr=boolean
  Constant : Constant  Value=0  OutDataTypeStr=fixdt(1,16,14)
  Real-Imag to Complex : RealImagToComplex
  Switch : Switch  Criteria=u2 ~= 0  SaturateOnIntegerOverflow=off  InputSameDT=off
  ctrl_gen : Subsystem
  data_out : Outport
  ctrl_out : Outport  Port=2
  wires:
  Real-Imag to Complex/1 -> Switch/3
  data_in/1 -> Switch/1
  ctrl_gen/2(ctrl_out) -> ctrl_out/1
  ctrl_gen/1(data_out) -> data_out/1
  select_valid/1 -> Switch/2, ctrl_gen/2(valid_in)
  Constant/1 -> Real-Imag to Complex/1, Real-Imag to Complex/2
  Switch/1 -> ctrl_gen/1(data_in)

== system rx2/process divide/transport_block3/Subsystem2 ==
  data_in : Inport
  select_valid : Inport  Port=2  OutDataTypeStr=boolean
  Constant : Constant  Value=0  OutDataTypeStr=fixdt(1,16,14)
  Real-Imag to Complex : RealImagToComplex
  Switch : Switch  Criteria=u2 ~= 0  SaturateOnIntegerOverflow=off  InputSameDT=off
  ctrl_gen : Subsystem
  data_out : Outport
  ctrl_out : Outport  Port=2
  wires:
  Real-Imag to Complex/1 -> Switch/3
  data_in/1 -> Switch/1
  ctrl_gen/2(ctrl_out) -> ctrl_out/1
  ctrl_gen/1(data_out) -> data_out/1
  select_valid/1 -> Switch/2, ctrl_gen/2(valid_in)
  Constant/1 -> Real-Imag to Complex/1, Real-Imag to Complex/2
  Switch/1 -> ctrl_gen/1(data_in)

== system rx2/process divide/transport_block3/Subsystem3 ==
  data_in : Inport
  select_valid : Inport  Port=2  OutDataTypeStr=boolean
  Constant : Constant  Value=0  OutDataTypeStr=fixdt(1,16,14)
  Real-Imag to Complex : RealImagToComplex
  Switch : Switch  Criteria=u2 ~= 0  SaturateOnIntegerOverflow=off  InputSameDT=off
  ctrl_gen : Subsystem
  data_out : Outport
  ctrl_out : Outport  Port=2
  wires:
  Switch/1 -> ctrl_gen/1(data_in)
  Constant/1 -> Real-Imag to Complex/2, Real-Imag to Complex/1
  select_valid/1 -> ctrl_gen/2(valid_in), Switch/2
  ctrl_gen/1(data_out) -> data_out/1
  ctrl_gen/2(ctrl_out) -> ctrl_out/1
  data_in/1 -> Switch/1
  Real-Imag to Complex/1 -> Switch/3

== system rx2/process divide/transport_block3/Subsystem4 ==
  data_in : Inport
  select_valid : Inport  Port=2  OutDataTypeStr=boolean
  Constant : Constant  Value=0  OutDataTypeStr=fixdt(1,16,14)
  Real-Imag to Complex : RealImagToComplex
  Switch : Switch  Criteria=u2 ~= 0  SaturateOnIntegerOverflow=off  InputSameDT=off
  ctrl_gen : Subsystem
  data_out : Outport
  ctrl_out : Outport  Port=2
  wires:
  Real-Imag to Complex/1 -> Switch/3
  data_in/1 -> Switch/1
  ctrl_gen/2(ctrl_out) -> ctrl_out/1
  ctrl_gen/1(data_out) -> data_out/1
  select_valid/1 -> Switch/2, ctrl_gen/2(valid_in)
  Constant/1 -> Real-Imag to Complex/1, Real-Imag to Complex/2
  Switch/1 -> ctrl_gen/1(data_in)

== system rx2/process divide/transport_block3/Subsystem5 ==
  data_in : Inport
  select_valid : Inport  Port=2  OutDataTypeStr=boolean
  Constant : Constant  Value=0  OutDataTypeStr=fixdt(1,16,14)
  Real-Imag to Complex : RealImagToComplex
  Switch : Switch  Criteria=u2 ~= 0  SaturateOnIntegerOverflow=off  InputSameDT=off
  ctrl_gen : Subsystem
  data_out : Outport
  ctrl_out : Outport  Port=2
  wires:
  Real-Imag to Complex/1 -> Switch/3
  data_in/1 -> Switch/1
  ctrl_gen/2(ctrl_out) -> ctrl_out/1
  ctrl_gen/1(data_out) -> data_out/1
  select_valid/1 -> Switch/2, ctrl_gen/2(valid_in)
  Constant/1 -> Real-Imag to Complex/1, Real-Imag to Complex/2
  Switch/1 -> ctrl_gen/1(data_in)

== system rx2/process divide/transport_block3/Subsystem6 ==
  data_in : Inport
  select_valid : Inport  Port=2  OutDataTypeStr=boolean
  Constant : Constant  Value=0  OutDataTypeStr=fixdt(1,16,14)
  Real-Imag to Complex : RealImagToComplex
  Switch : Switch  Criteria=u2 ~= 0  SaturateOnIntegerOverflow=off  InputSameDT=off
  ctrl_gen : Subsystem
  data_out : Outport
  ctrl_out : Outport  Port=2
  wires:
  Real-Imag to Complex/1 -> Switch/3
  data_in/1 -> Switch/1
  ctrl_gen/2(ctrl_out) -> ctrl_out/1
  ctrl_gen/1(data_out) -> data_out/1
  select_valid/1 -> Switch/2, ctrl_gen/2(valid_in)
  Constant/1 -> Real-Imag to Complex/1, Real-Imag to Complex/2
  Switch/1 -> ctrl_gen/1(data_in)

== system rx2/process divide/transport_block3/Subsystem7 ==
  data_in : Inport
  select_valid : Inport  Port=2  OutDataTypeStr=boolean
  Constant : Constant  Value=0  OutDataTypeStr=fixdt(1,16,14)
  Real-Imag to Complex : RealImagToComplex
  Switch : Switch  Criteria=u2 ~= 0  SaturateOnIntegerOverflow=off  InputSameDT=off
  ctrl_gen : Subsystem
  data_out : Outport
  ctrl_out : Outport  Port=2
  wires:
  Real-Imag to Complex/1 -> Switch/3
  data_in/1 -> Switch/1
  ctrl_gen/2(ctrl_out) -> ctrl_out/1
  ctrl_gen/1(data_out) -> data_out/1
  select_valid/1 -> Switch/2, ctrl_gen/2(valid_in)
  Constant/1 -> Real-Imag to Complex/1, Real-Imag to Complex/2
  Switch/1 -> ctrl_gen/1(data_in)
